simulink model "cubli_XYZ_extensive_simulations"  (R2016a)
settings: Solver=VariableStepAuto  StartTime=0.0  StopTime=10  FixedStep=0.001  RelTol=1e-3
values from neighbouring files (symbols this model uses):
  a = 0.15    [init.m]
  M = 2.5    [init.m]    (also in skew.m = [0 -z y)
  m = 0.204    [init.m]
  s = size(delta_i)    [accessibility_test.m]    (also in observability_test.m = size(delta_i,1))
  state0 = get_equilibrium(0, -pi/4, pi/2, f, state)    [init.m]
undefined symbols (not defined in the file or in its folder): X, Y, Z
libraries: sm_lib x15, nesl_utility x13
(part 9 of 9)

== matlab function cubli_XYZ_extensive_simulations/Cubli/Cubli/Wrap between +-pi ==
  data: u input; y output
function y = wrap(u)
coder.extrinsic('wrapToPi');

y = [0;0;0];
y = wrapToPi(u);

== matlab function cubli_XYZ_extensive_simulations/Cubli/Wrap between +-pi ==
  data: u input; y output
function y = wrap(u)
coder.extrinsic('wrapToPi');

y = [0;0;0];
y = wrapToPi(u);

== matlab function cubli_XYZ_extensive_simulations/Cubli/Reference/Wrap between +-pi ==
  data: u input; y output
function y = wrap(u)
coder.extrinsic('wrapToPi');

y = [0;0;0];
y = wrapToPi(u);

== matlab function cubli_XYZ_extensive_simulations/Cubli/MATLAB Function ==
  data: error input; unstable output; max_error input
function unstable = fcn(error, max_error)
unstable = 0;

if (error(1) > max_error || error(2) > max_error || error(3) > max_error)
    unstable = 1;
end

== matlab function cubli_XYZ_extensive_simulations/Cubli/Cubli/MATLAB Function ==
  data: velocities input; y output; time input; switch_time input
function y = fcn(velocities, time, switch_time)
persistent final_velocity;

if isempty(final_velocity)
     final_velocity = [0, 0, 0];
end

if time < switch_time
    final_velocity = velocities';
end
    y = final_velocity;
end
